simulink model "Final_6_9_21_simu"  (R2021a)
settings: Solver=VariableStepAuto  StartTime=0.0  StopTime=50.0  RelTol=1e-3
values from neighbouring files (symbols this model uses):
  ue = 2    [Final_6_9_21.m]
  xe = [x1e; x2e]    [Final_6_9_21.m]
  ye = 8    [Final_6_9_21.m]
libraries: cstblocks x1
settings Model: Creator=Santiago  LastModifiedBy=Santiago

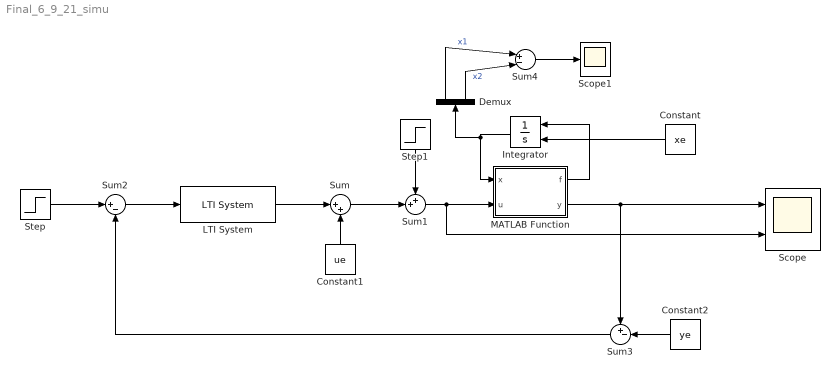
== system Final_6_9_21_simu ==
  Constant : Constant  Value=xe
  Constant1 : Constant  Value=ue
  Constant2 : Constant  Value=ye
  Demux : Demux  Outputs=2
  Integrator : Integrator  InitialConditionSource=external
  LTI System : cstblocks/LTI System  sys=C_dig  IC=[]
  MATLAB Function : MATLAB Function  TreatAsAtomicUnit=on
  Scope : Scope  NumInputPorts=2
  Scope1 : Scope
  Step : Step  After=-4  SampleTime=0
  Step1 : Step  Time=5  After=0.5*ue  SampleTime=0
  Sum : Sum  Inputs=|++
  Sum1 : Sum  Inputs=++|
  Sum2 : Sum  Inputs=|+-
  Sum3 : Sum  Inputs=+-|
  Sum4 : Sum  Inputs=|+-|
  wires:
  Constant/1 -> Integrator/2
  Integrator/1 -> Demux/1, MATLAB Function/1(x)
  MATLAB Function/1(f) -> Integrator/1
  Constant1/1 -> Sum/2
  LTI System/1 -> Sum/1
  Sum/1 -> Sum1/2
  Sum1/1 -> Scope/2, MATLAB Function/2(u)
  MATLAB Function/2(y) -> Sum3/1, Scope/1
  Constant2/1 -> Sum3/2
  Sum3/1 -> Sum2/2
  Sum2/1 -> LTI System/1
  Step/1 -> Sum2/1
  Step1/1 -> Sum1/1
  Demux/2 -> Sum4/2  "x2"
  Demux/1 -> Sum4/1  "x1"
  Sum4/1 -> Scope1/1

== matlab function Final_6_9_21_simu/MATLAB Function ==
  data: x input; f output; u input; y output
function [f, y] = fcn(x, u)
x1 = x(1);
x2 = x(2);

f1 = -sqrt(abs(x1 - x2)) + u;
f2 = sqrt(abs(x1 - x2)) - sqrt(abs(x2));
f = [f1; f2];

y = x1;
